simulink model "DCFastCharger"  (R2023b)
settings: Solver=ode23t  StartTime=0.0  StopTime=simulation.simTime  MaxStep=1/(5*inverter.SwitchFrequency)  RelTol=1e-3  AbsTol=1e-3
PreLoadFcn:
  | run('DCFastChargerData.mlx');
undefined symbols (not defined in the file or in its folder): battery, inverter, rectifier
libraries: nesl_utility x34, fl_lib x22, ee_lib x14, eePwmGenerator x2, eeTransforms x2, batteryecm_lib x1, eeSinusoidalMeasurement x1, slpidlib x1, eePwmGeneratorThreeLevel x1, eePwmGeneratorTwoLevel x1, simulink_extras x1
(part 3 of 3)

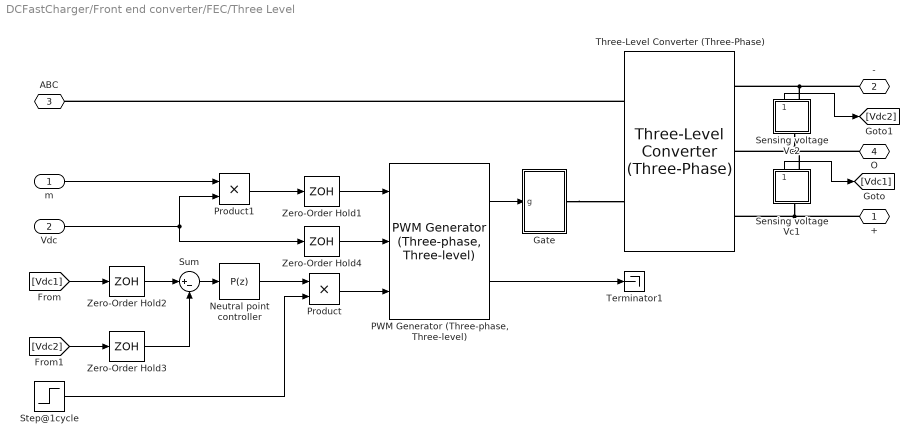
== system DCFastCharger/Front end converter/FEC/Three Level ==
  m : Inport
  Vdc : Inport  Port=2
  Gate : Subsystem
  Neutral point controller : slpidlib/PID Controller  Controller=P  Form=Parallel  TimeDomain=Discrete-time  UseExternalTs=off  SampleTime=-1  IntegratorMethod=Forward Euler  FilterMethod=Forward Euler  ControllerParametersSource=internal  P=0.001  I=80/2  UseKiTs=off  D=0  N=100  UseFilter=on  TunerSelectOption=Transfer Function Based (PID Tuner App)  ZeroCross=off  InitialConditionSource=internal  InitialConditionForIntegrator=0  InitialConditionForFilter=0  DifferentiatorICPrevScaledInput=0  ExternalReset=none  TrackingMode=off  Kt=1  LimitOutput=on  SatLimitsSource=internal  UpperSaturationLimit=1  LowerSaturationLimit=-1  LinearizeAsGain=on  AntiWindupMode=back-calculation  Kb=1000  LimitIntegrator=off  UpperIntegratorSaturationLimit=inf  LowerIntegratorSaturationLimit=-inf  POutMin=[]  POutMax=[]  IOutMin=[]  IOutMax=[]  DOutMin=[]  DOutMax=[]  NOutMin=[]  NOutMax=[]  SumOutMin=[]  SumOutMax=[]  SaturationOutMin=[]  SaturationOutMax=[]  PParamMin=[]  PParamMax=[]  IParamMin=[]  IParamMax=[]  DParamMin=[]  DParamMax=[]  NParamMin=[]  NParamMax=[]  KbParamMin=[]  KbParamMax=[]  KtParamMin=[]  KtParamMax=[]  KbOutMin=[]  KbOutMax=[]  KtOutMin=[]  KtOutMax=[]  IntegratorOutMin=[]  IntegratorOutMax=[]  FilterOutMin=[]  FilterOutMax=[]  SumI1OutMin=[]  SumI1OutMax=[]  SumI2OutMin=[]  SumI2OutMax=[]  SumI3OutMin=[]  SumI3OutMax=[]  SumI4OutMin=[]  SumI4OutMax=[]  SumDOutMin=[]  SumDOutMax=[]  DifferentiatorOutMin=[]  DifferentiatorOutMax=[]  FilterDiffOutCoefMin=[]  FilterDiffOutCoefMax=[]  ReciprocalOutMin=[]  ReciprocalOutMax=[]  SumDenOutMin=[]  SumDenOutMax=[]  SumNumOutMin=[]  SumNumOutMax=[]  DivideOutMin=[]  DivideOutMax=[]  UdiffTsProdOutMin=[]  UdiffTsProdOutMax=[]  NTsProdOutMin=[]  NTsProdOutMax=[]  UintegralTsProdOutMin=[]  UintegralTsProdOutMax=[]  UngainTsProdOutMin=[]  UngainTsProdOutMax=[]  ClampingZeroOutDataTypeStr=Inherit: Inherit via back propagation  ClampingZeroOutMin=[]  ClampingZeroOutMax=[]  FilterDenConstantOutDataTypeStr=Inherit: Inherit via back propagation  FilterDenConstantOutMin=[]  FilterDenConstantOutMax=[]  PCopyOutDataTypeStr=Inherit: Inherit via back propagation  PCopyOutMin=[]  PCopyOutMax=[]  NCopyOutDataTypeStr=Inherit: Inherit via back propagation  NCopyOutMin=[]  NCopyOutMax=[]  IntegratorContinuousStateAttributes=''  IntegratorStateMustResolveToSignalObject=off  IntegratorRTWStateStorageClass=Auto  FilterContinuousStateAttributes=''  FilterStateMustResolveToSignalObject=off  FilterRTWStateStorageClass=Auto  ParallelPVariant=InternalParameters  IdealPVariant=Disabled  IVariant=Disabled  DVariant=Disabled  IntegratorVariant=Disabled  SatVariant=Enabled  AWVariant=Disabled  PCopyVariant=Disabled  TRVariant=Disabled  FdbkBlocksVariant=Forward  IdealPFdbkVariant=Disabled  SatFdbkVariant=Disabled  DerivativeFilterVariant=Disabled  NVariant=Disabled  NCopyVariant=Disabled_SignalSpec  FilterICVariant=Disabled  IntegratorICVariant=Disabled  ExternalResetVariant=Disabled  TRSumVariant=Passthrough  SumFdbkVariant=Disabled  SumVariant=Passthrough_P  TsampFilterVariant=InternalTs  TsampNgainVariant=Passthrough  TsampIntegralVariant=Disabled_SignalSpec  ExternalSaturationOutDataTypeStr=Inherit: Same as second input
  "PWM Generator (Three-phase, Three-level)" : eePwmGeneratorThreeLevel/PWM Generator (Three-phase, Three-level)  CPWMMode=SPWM: sinusoidal PWM  fsw=rectifier.SwitchFrequency  Ts=1/(10*rectifier.SwitchFrequency)
      settings: SamplingMode=Natural
  Product : Product
  Product1 : Product
  Sensing voltage Vc1 : Subsystem
      mask Display: disp('Vdc1')
  Sensing voltage Vc2 : Subsystem
      mask Display: disp('Vdc2')
  Step@1cycle : Step  Time=1/rectifier.SystemFrequency  SampleTime=1/(10*rectifier.SwitchFrequency)
  Sum : Sum  Inputs=|+-
  Terminator1 : Terminator
  Three-Level Converter (Three-Phase) : ee_lib/Semiconductors & Converters/Converters/Three-Level Converter (Three-Phase)  port_option=ee.enum.threePhasePort.composite  device_type=2  Vf=0.8 V  Ron=0.001 Ohm  Rds=0.001 Ohm  Goff=1e-6 1/Ohm  Vth=0.2 V  Vgt=1 V  Vgt_off=-1 V  Ih=1 A  K=0  diode_param=2  diode_Vf=0.8 V  diode_Ron=0.001 Ohm  diode_Goff=1e-5 1/Ohm  diode_C=50 nF  diode_iRM=-235 A  diode_iF=300 A  diode_idot=-50 A/us  diode_trr_param=1  diode_trr_factor=3  diode_trr=15 us  diode_Qrr=1500 s*uA  snubber_type=0  Cs=1e-7 F  Rs=0.1 Ohm
      settings: InternalSimscapePortConfiguration="{\"Bottom\":[],\"Left\":[{\"id\":\"G\",\"label\":\"G\",\"type\":\"foundation.electrical.twenty_four_phase\"},{\"id\":\"N\",\"label\":\"~\",\"type\":\"foundation.electrical.three_phase\"}],\"Right\":[{\"id\":\"p\",\"label\":\"+\",\"type\":\"foundation.electrical.electrical\"},{\"id\":\"z\",\"label\":\"0\",\"type\":\"foundation.electrical.electrical\"},{\"id\":\"n\",\"label\":\"-\",\"type\":\"foundation.electrical.electrical\"}],\"Top\":[]}"
  Zero-Order Hold1 : ZeroOrderHold  SampleTime=1/(10*rectifier.SwitchFrequency)
  Zero-Order Hold2 : ZeroOrderHold  SampleTime=1/(5*rectifier.SwitchFrequency)
  Zero-Order Hold3 : ZeroOrderHold  SampleTime=1/(5*rectifier.SwitchFrequency)
  Zero-Order Hold4 : ZeroOrderHold  SampleTime=1/(10*rectifier.SwitchFrequency)
  + : PMIOPort  Side=Right
  - : PMIOPort  Port=2  Side=Right
  ABC : PMIOPort  Port=3  Side=Left
  O : PMIOPort  Port=4  Side=Right
  wires:
  Sum/1 -> Neutral point controller/1
  Vdc/1 -> Zero-Order Hold4/1, Product1/2
  m/1 -> Product1/1
  Zero-Order Hold2/1 -> Sum/1
  Zero-Order Hold3/1 -> Sum/2
  Zero-Order Hold1/1 -> "PWM Generator (Three-phase, Three-level)"/1
  Zero-Order Hold4/1 -> "PWM Generator (Three-phase, Three-level)"/2
  "PWM Generator (Three-phase, Three-level)"/2 -> Terminator1/1
  Product1/1 -> Zero-Order Hold1/1
  [Vdc1] -> Zero-Order Hold2/1
  Step@1cycle/1 -> Product/2
  [Vdc2] -> Zero-Order Hold3/1
  Neutral point controller/1 -> Product/1
  Product/1 -> "PWM Generator (Three-phase, Three-level)"/3
  "PWM Generator (Three-phase, Three-level)"/1 -> Gate/1(g)
  Sensing voltage Vc1/1(Out1) -> [Vdc1]
  Sensing voltage Vc2/1(Out1) -> [Vdc2]
  connections:
  Sensing voltage Vc2/LConn1 -- Sensing voltage Vc1/RConn1 -- O/RConn1 -- Three-Level Converter (Three-Phase)/RConn2
  -/RConn1 -- Three-Level Converter (Three-Phase)/RConn3 -- Sensing voltage Vc2/RConn1
  +/RConn1 -- Three-Level Converter (Three-Phase)/RConn1 -- Sensing voltage Vc1/LConn1
  Three-Level Converter (Three-Phase)/LConn2 -- ABC/RConn1
  Gate/RConn1 -- Three-Level Converter (Three-Phase)/LConn1

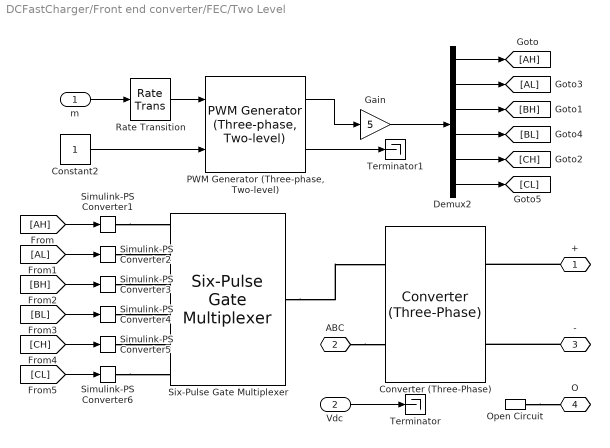
== system DCFastCharger/Front end converter/FEC/Two Level ==
  m : Inport
  Vdc : Inport  Port=2
  Constant2 : Constant
  Converter (Three-Phase) : ee_lib/Semiconductors & Converters/Converters/Converter (Three-Phase)  port_option=ee.enum.threePhasePort.composite  device_type=ee.enum.converters.switchingdevice.ideal  K=0  Vf=0.8 V  Ron=0.001 Ohm  Rds=0.001 Ohm  Goff=1e-6 1/Ohm  Vgt=1 V  Vgt_off=-1 V  Ih=1 A  Vth=0.5 V  diode_param=ee.enum.converters.protectiondiode.nodynamics  diode_Vf=0.06 V  diode_Ron=0.001 Ohm  diode_Goff=1e-5 1/Ohm  diode_C=50 nF  diode_iRM=-235 A  diode_iF=300 A  diode_idot=-50 A/us  diode_trr_param=ee.enum.converters.diodetrr.trr_factor  diode_trr_factor=3  diode_trr=15 us  diode_Qrr=1500 s*uA  snubber_type=ee.enum.converters.snubber.exclude  Cs=1e-7 F  Rs=0.1 Ohm
  Demux2 : Demux  Outputs=6
  Gain : Gain  Gain=5
  Open Circuit : fl_lib/Electrical/Electrical Elements/Open Circuit  v_specify=off  v_priority=None  v=0 V  v_nominal_specify=off  v_nominal_unit=V  v_nominal_value=1
  "PWM Generator (Three-phase, Two-level)" : eePwmGeneratorTwoLevel/PWM Generator (Three-phase, Two-level)  PWMMode=Continuous PWM (CPWM)  CPWMMode=SVM: space vector modulation  DPWMMode=60 DPWM: 60 degree discontinuous PWM  fsw=rectifier.SwitchFrequency  Ts=rectifier.VoltageSensorT
  Rate Transition : RateTransition  OutPortSampleTime=rectifier.VoltageSensorT
  Simulink-PS Converter{1..6} (6 alike) : nesl_utility/Simulink-PS Converter  PhysicalDomain=network_engine_domain  SubClassName=ps_input  LeftPortType=input  RightPortType=output  PseudoPeriodic=off  Frequencies=[]  NoiseDistribution=none  NoiseParameters=[]  Unit=1  AffineConversion=off  FilteringAndDerivatives=provide  SimscapeFilterOrder=1  InputFilterTimeConstant=0.001  UdotUserProvided=0
  Six-Pulse Gate Multiplexer : ee_lib/Semiconductors & Converters/Converters/Six-Pulse Gate Multiplexer  port_option=ee.enum.controlport.ps
  Terminator : Terminator
  Terminator1 : Terminator
  + : PMIOPort  Side=Right
  ABC : PMIOPort  Port=2  Side=Left
  - : PMIOPort  Port=3  Side=Right
  O : PMIOPort  Port=4  Side=Right
  wires:
  [AH] -> Simulink-PS Converter1/1
  [CL] -> Simulink-PS Converter6/1
  [AL] -> Simulink-PS Converter2/1
  [BL] -> Simulink-PS Converter4/1
  [CH] -> Simulink-PS Converter5/1
  [BH] -> Simulink-PS Converter3/1
  Gain/1 -> Demux2/1
  Rate Transition/1 -> "PWM Generator (Three-phase, Two-level)"/1
  Demux2/2 -> [AL]
  Demux2/1 -> [AH]
  Demux2/5 -> [CH]
  Demux2/3 -> [BH]
  "PWM Generator (Three-phase, Two-level)"/1 -> Gain/1
  Demux2/4 -> [BL]
  Demux2/6 -> [CL]
  Constant2/1 -> "PWM Generator (Three-phase, Two-level)"/2
  m/1 -> Rate Transition/1
  Vdc/1 -> Terminator/1
  "PWM Generator (Three-phase, Two-level)"/2 -> Terminator1/1
  connections:
  ABC/RConn1 -- Converter (Three-Phase)/LConn2
  Simulink-PS Converter1/RConn1 -- Six-Pulse Gate Multiplexer/LConn1
  Simulink-PS Converter2/RConn1 -- Six-Pulse Gate Multiplexer/LConn2
  Simulink-PS Converter3/RConn1 -- Six-Pulse Gate Multiplexer/LConn3
  Simulink-PS Converter4/RConn1 -- Six-Pulse Gate Multiplexer/LConn4
  Simulink-PS Converter5/RConn1 -- Six-Pulse Gate Multiplexer/LConn5
  Simulink-PS Converter6/RConn1 -- Six-Pulse Gate Multiplexer/LConn6
  Six-Pulse Gate Multiplexer/RConn1 -- Converter (Three-Phase)/LConn1
  +/RConn1 -- Converter (Three-Phase)/RConn1
  -/RConn1 -- Converter (Three-Phase)/RConn2
  Open Circuit/LConn1 -- O/RConn1

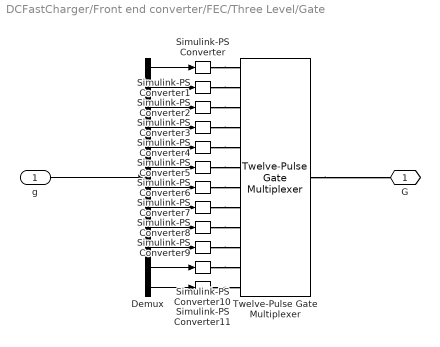
== system DCFastCharger/Front end converter/FEC/Three Level/Gate ==
  g : Inport
  Demux : Demux  Outputs=12
  Simulink-PS Converter{,1..11} (12 alike) : nesl_utility/Simulink-PS Converter  PhysicalDomain=network_engine_domain  SubClassName=ps_input  LeftPortType=input  RightPortType=output  PseudoPeriodic=off  Frequencies=[]  NoiseDistribution=none  NoiseParameters=[]  Unit=1  AffineConversion=off  FilteringAndDerivatives=zero  SimscapeFilterOrder=1  InputFilterTimeConstant=0.001  UdotUserProvided=1
  Twelve-Pulse Gate Multiplexer : ee_lib/Semiconductors & Converters/Converters/Twelve-Pulse Gate Multiplexer  port_option=ee.enum.controlport.ps
      settings: InternalSimscapePortConfiguration="{\"Bottom\":[],\"Left\":[{\"id\":\"Ga1_ps\",\"label\":\"Ga(1)\",\"type\":\"input\"},{\"id\":\"Ga2_ps\",\"label\":\"Ga(2)\",\"type\":\"input\"},{\"id\":\"Ga3_ps\",\"label\":\"Ga(3)\",\"type\":\"input\"},{\"id\":\"Ga4_ps\",\"label\":\"Ga(4)\",\"type\":\"input\"},{\"id\":\"Gb1_ps\",\"label\":\"Gb(1)\",\"type\":\"input\"},{\"id\":\"Gb2_ps\",\"label\":\"Gb(2)\",\"type\":\"input\"},{\"id\":\"Gb3_ps\",\"label\":\"Gb(3)\",\"type\":\"input\"},{\"id\":\"Gb4_ps\",\"label\":\"Gb(4)\",\"type\":\"input\"},{\"id\":\"Gc1_ps\",\"label\":\"Gc(1)\",\"type\":\"input\"},{\"id\":\"Gc2_ps\",\"label\":\"Gc(2)\",\"type\":\"input\"},{\"id\":\"Gc3_ps\",\"label\":\"Gc(3)\",\"type\":\"input\"},{\"id\":\"Gc4_ps\",\"label\":\"Gc(4)\",\"type\":\"input\"}],\"Right\":[{\"id\":\"p\",\"label\":\"G\",\"type\":\"foundation.electrical.twenty_four_phase\"}],\"Top\":[]}"
  G : PMIOPort  Side=Right
  wires:
  g/1 -> Demux/1
  Demux/5 -> Simulink-PS Converter4/1
  Demux/10 -> Simulink-PS Converter9/1
  Demux/2 -> Simulink-PS Converter1/1
  Demux/9 -> Simulink-PS Converter8/1
  Demux/12 -> Simulink-PS Converter11/1
  Demux/3 -> Simulink-PS Converter2/1
  Demux/7 -> Simulink-PS Converter6/1
  Demux/6 -> Simulink-PS Converter5/1
  Demux/4 -> Simulink-PS Converter3/1
  Demux/1 -> Simulink-PS Converter/1
  Demux/11 -> Simulink-PS Converter10/1
  Demux/8 -> Simulink-PS Converter7/1
  connections:
  Simulink-PS Converter10/RConn1 -- Twelve-Pulse Gate Multiplexer/LConn11
  Simulink-PS Converter8/RConn1 -- Twelve-Pulse Gate Multiplexer/LConn9
  Simulink-PS Converter/RConn1 -- Twelve-Pulse Gate Multiplexer/LConn1
  Simulink-PS Converter11/RConn1 -- Twelve-Pulse Gate Multiplexer/LConn12
  Simulink-PS Converter3/RConn1 -- Twelve-Pulse Gate Multiplexer/LConn4
  Simulink-PS Converter2/RConn1 -- Twelve-Pulse Gate Multiplexer/LConn3
  Simulink-PS Converter4/RConn1 -- Twelve-Pulse Gate Multiplexer/LConn5
  Simulink-PS Converter1/RConn1 -- Twelve-Pulse Gate Multiplexer/LConn2
  Twelve-Pulse Gate Multiplexer/RConn1 -- G/RConn1
  Simulink-PS Converter5/RConn1 -- Twelve-Pulse Gate Multiplexer/LConn6
  Simulink-PS Converter9/RConn1 -- Twelve-Pulse Gate Multiplexer/LConn10
  Simulink-PS Converter6/RConn1 -- Twelve-Pulse Gate Multiplexer/LConn7
  Simulink-PS Converter7/RConn1 -- Twelve-Pulse Gate Multiplexer/LConn8

== system DCFastCharger/Front end converter/FEC/Three Level/Sensing voltage Vc1 ==
  PS-Simulink Converter : nesl_utility/PS-Simulink Converter  PhysicalDomain=network_engine_domain  SubClassName=ps_output  LeftPortType=input  RightPortType=output  PseudoPeriodic=off  Frequencies=[]  VectorFormat=1-D array  Unit=1  AffineConversion=off
  Sensor dynamics : TransferFcn  Numerator=rectifier.VoltageSensorG  Denominator=[rectifier.VoltageSensorT 1]
  Vc1 : fl_lib/Electrical/Electrical Sensors/Voltage Sensor
  + : PMIOPort  Side=Left
  - : PMIOPort  Port=2  Side=Right
  Out1 : Outport
  wires:
  PS-Simulink Converter/1 -> Sensor dynamics/1
  Sensor dynamics/1 -> Out1/1
  connections:
  Vc1/RConn2 -- -/RConn1
  Vc1/LConn1 -- +/RConn1
  PS-Simulink Converter/LConn1 -- Vc1/RConn1

== system DCFastCharger/Front end converter/FEC/Three Level/Sensing voltage Vc2 ==
  PS-Simulink Converter : nesl_utility/PS-Simulink Converter  PhysicalDomain=network_engine_domain  SubClassName=ps_output  LeftPortType=input  RightPortType=output  PseudoPeriodic=off  Frequencies=[]  VectorFormat=1-D array  Unit=1  AffineConversion=off
  Sensor dynamics : TransferFcn  Numerator=rectifier.VoltageSensorG  Denominator=[rectifier.VoltageSensorT 1]
  Vc2 : fl_lib/Electrical/Electrical Sensors/Voltage Sensor
  Conn1 : PMIOPort  Side=Left
  Conn3 : PMIOPort  Port=2  Side=Right
  Out1 : Outport
  wires:
  Sensor dynamics/1 -> Out1/1
  PS-Simulink Converter/1 -> Sensor dynamics/1
  connections:
  Vc2/RConn2 -- Conn3/RConn1
  Vc2/LConn1 -- Conn1/RConn1
  PS-Simulink Converter/LConn1 -- Vc2/RConn1
